simulink model "wearg"  (R2018a)
settings: Solver=VariableStepAuto  StartTime=0.0  StopTime=10.0  RelTol=1e-3
settings Model: Creator=9920103168  LastModifiedBy=9920103168

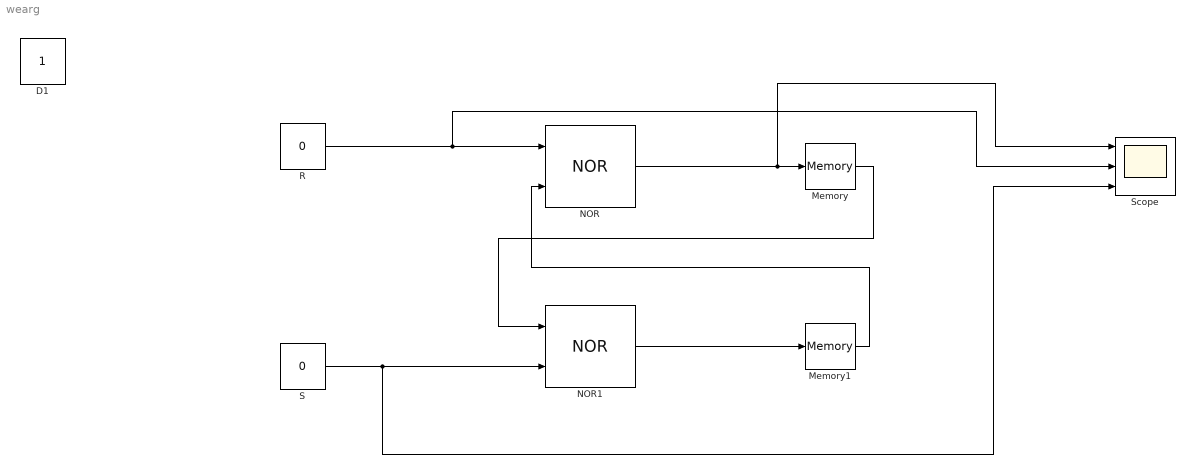
== system wearg ==
  "D1 " : Constant
  Memory : Memory
  Memory1 : Memory
  NOR : Logic  Operator=NOR  IconShape=distinctive  AllPortsSameDT=off  OutDataTypeStr=boolean
  NOR1 : Logic  Operator=NOR  IconShape=distinctive  AllPortsSameDT=off  OutDataTypeStr=boolean
  R : Constant  Value=0
  S : Constant  Value=0
  Scope : Scope  NumInputPorts=3
  wires:
  NOR/1 -> Scope/1, Memory/1
  S/1 -> Scope/3, NOR1/2
  NOR1/1 -> Memory1/1
  Memory1/1 -> NOR/2
  Memory/1 -> NOR1/1
  R/1 -> Scope/2, NOR/1
